simulink subsystem "Plant_with_changing_dynamics"  (R2022a)
settings: Solver=VariableStepAuto  StartTime=0.0  StopTime=10.0  RelTol=1e-3
settings Model: Creator=intel  LastModifiedBy=intel

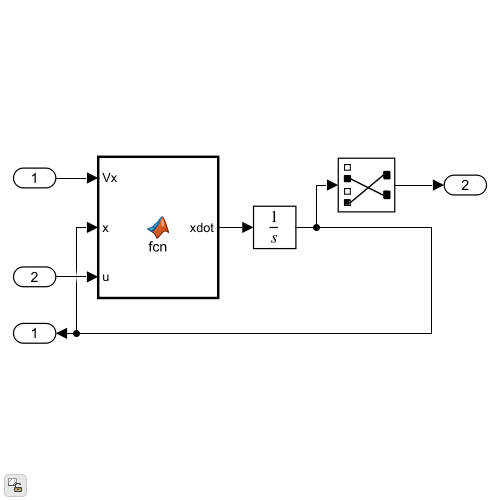
[thumbnail: Simulink's stored preview of the top-level diagram]
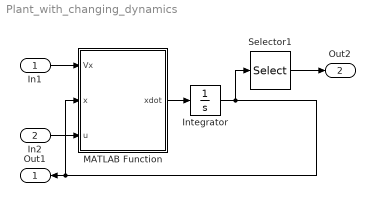
== system Plant_with_changing_dynamics ==
  In1 : Inport
  In2 : Inport  Port=2
  Integrator : Integrator
  MATLAB Function : MATLAB Function  TreatAsAtomicUnit=on
  Selector1 : Selector  InputPortWidth=4  IndexOptions=Index vector (dialog)  Indices=[4 2]  OutputSizes=1
  Out1 : Outport  VectorParamsAs1DForOutWhenUnconnected=off
  Out2 : Outport  Port=2  VectorParamsAs1DForOutWhenUnconnected=off
  wires:
  In2/1 -> MATLAB Function/3(u)
  In1/1 -> MATLAB Function/1(Vx)
  Integrator/1 -> Out1/1, MATLAB Function/2(x), Selector1/1
  MATLAB Function/1(xdot) -> Integrator/1
  Selector1/1 -> Out2/1

== matlab function Plant_with_changing_dynamics/MATLAB Function ==
  data: Vx input; x input size=[4,1]; u input; xdot output size=[4,1]
function xdot = fcn(Vx,x,u)

% Model parameters
m = 1575;
Iz = 2875;
lf = 1.2;
lr = 1.6;
Cf = 19000;
Cr = 33000;

% Continuous-time model
A = [-(2*Cf+2*Cr)/m/Vx, 0, -Vx-(2*Cf*lf-2*Cr*lr)/m/Vx, 0;
     0, 0, 1, 0;
     -(2*Cf*lf-2*Cr*lr)/Iz/Vx, 0, -(2*Cf*lf^2+2*Cr*lr^2)/Iz/Vx, 0;
     1, Vx, 0, 0];
B = [2*Cf/m 0 2*Cf*lf/Iz 0]';   
C = [0 0 0 1; 0 1 0 0];
D = zeros(2,1);
xdot = A*x + B*u;
%y = C*x + D*u;
